simulink library "accelerometers"  (R2023b)
settings: Solver=VariableStepAuto  StartTime=0.0  StopTime=10.0  RelTol=1e-3
values from neighbouring files (symbols this model uses):
  acc_dynamic = 2*9.81    (= 19.62)    [sim_cfg.m]
  acc_freq = 100    [sim_cfg.m]
  acc_noise = 0.008*9.81    (= 0.07848)    [sim_cfg.m]
  acc_non_orthogonality = acc_axis_alignement*acc_non_orthogonality    [sim_cfg.m]
  gravity = 9.81+rand()*0.005    [sim_cfg.m]
libraries: simulink x1
settings Model: Creator=robin  LastModifiedBy=robin

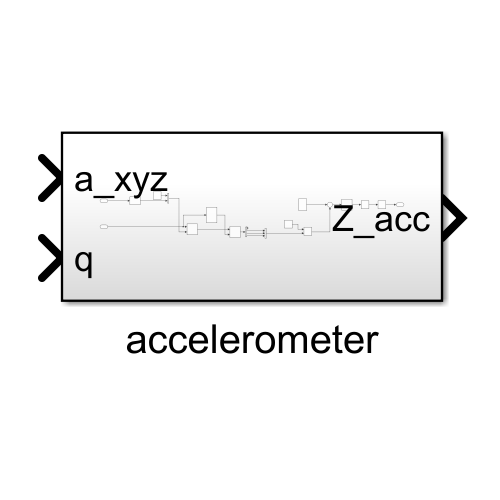
[thumbnail: Simulink's stored preview of the top-level diagram]
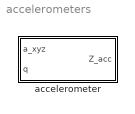
== system accelerometers ==
  accelerometer : Subsystem

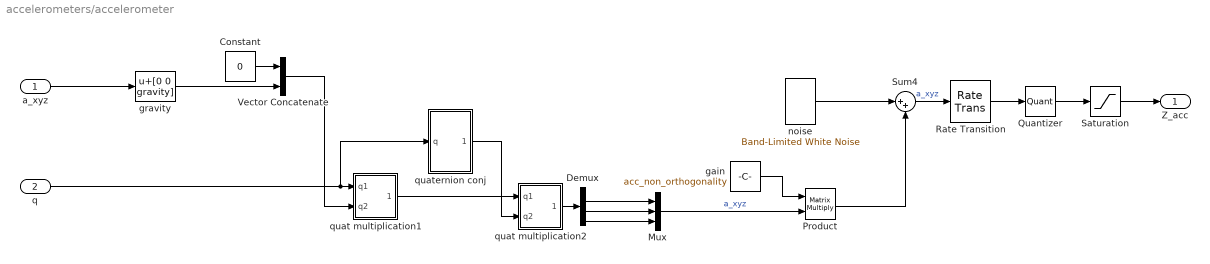
== system accelerometers/accelerometer ==
  a_xyz : Inport
  q : Inport  Port=2
  Constant : Constant  Value=0
  Demux : Demux
  Mux : Mux  Inputs=3
  Product : Product  Multiplication=Matrix(*)
  Quantizer : Quantizer  QuantizationInterval=acc_res
  Rate Transition : RateTransition  OutPortSampleTime=1/acc_freq
  Saturation : Saturate  UpperLimit=acc_dynamic  LowerLimit=-acc_dynamic
  Sum4 : Sum  Inputs=|++
  Vector Concatenate : Concatenate
  gain : Constant  Value=acc_non_orthogonality
  gravity : Bias  Bias=[0 0 gravity]  SaturateOnIntegerOverflow=off
  noise : simulink/Sources/Band-Limited White Noise  Cov=[2*(2*pi*acc_noise/acc_freq)^2 2*(2*pi*acc_noise/acc_freq)^2 2*(2*pi*acc_noise/acc_freq)^2]  Ts=1/acc_freq  seed=[randi(1000) randi(1000) randi(1000)]  VectorParams1D=off
  quat multiplication1 : Subsystem
  quat multiplication2 : Subsystem
  quaternion conj : Subsystem
  Z_acc : Outport
  wires:
  q/1 -> quat multiplication1/1(q1), quaternion conj/1(q)
  Sum4/1 -> Rate Transition/1  "a_xyz"
  Constant/1 -> Vector Concatenate/1
  Vector Concatenate/1 -> quat multiplication1/2(q2)
  gravity/1 -> Vector Concatenate/2
  quaternion conj/1(q conj) -> quat multiplication2/2(q2)
  quat multiplication1/1(q1*q2) -> quat multiplication2/1(q1)
  a_xyz/1 -> gravity/1
  quat multiplication2/1(q1*q2) -> Demux/1
  Demux/2 -> Mux/1
  Demux/3 -> Mux/2
  Demux/4 -> Mux/3
  gain/1 -> Product/1
  noise/1 -> Sum4/1
  Mux/1 -> Product/2  "a_xyz"
  Saturation/1 -> Z_acc/1
  Rate Transition/1 -> Quantizer/1
  Quantizer/1 -> Saturation/1
  Product/1 -> Sum4/2

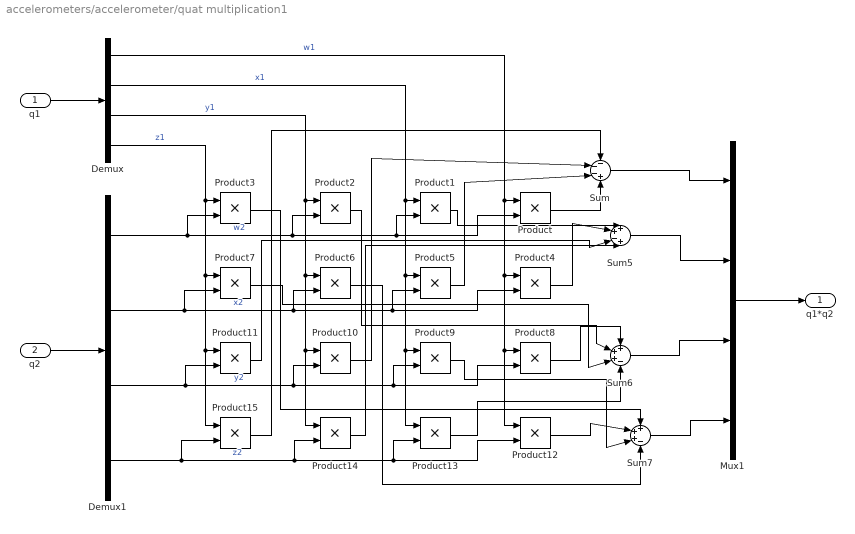
== system accelerometers/accelerometer/quat multiplication1 ==
  q1 : Inport
  q2 : Inport  Port=2
  Demux : Demux
  Demux1 : Demux
  Mux1 : Mux
  Product{,1..15} (16 alike) : Product
  Sum : Sum  Inputs=---+
  Sum5 : Sum  Inputs=++-+
  Sum6 : Sum  Inputs=+++-
  Sum7 : Sum  Inputs=+++-
  q1*q2 : Outport
  wires:
  Sum5/1 -> Mux1/2
  Product/1 -> Sum/4
  Product9/1 -> Sum7/3
  Demux/1 -> Product12/1, Product8/1, Product4/1, Product/1  "w1"
  Demux1/3 -> Product8/2, Product9/2, Product10/2, Product11/2  "y2"
  Demux/2 -> Product13/1, Product9/1, Product5/1, Product1/1  "x1"
  Product6/1 -> Sum7/4
  Product4/1 -> Sum5/2
  Demux1/1 -> Product/2, Product1/2, Product2/2, Product3/2  "w2"
  Sum/1 -> Mux1/1
  Product3/1 -> Sum7/1
  Product15/1 -> Sum/1
  Product1/1 -> Sum5/1
  Product2/1 -> Sum6/2
  Demux/4 -> Product15/1, Product11/1, Product7/1, Product3/1  "z1"
  Sum6/1 -> Mux1/3
  Demux1/2 -> Product4/2, Product5/2, Product6/2, Product7/2  "x2"
  Demux1/4 -> Product12/2, Product13/2, Product14/2, Product15/2  "z2"
  Product14/1 -> Sum5/4
  Mux1/1 -> q1*q2/1
  Sum7/1 -> Mux1/4
  Demux/3 -> Product14/1, Product10/1, Product6/1, Product2/1  "y1"
  Product13/1 -> Sum6/4
  Product8/1 -> Sum6/1
  q2/1 -> Demux1/1
  q1/1 -> Demux/1
  Product11/1 -> Sum5/3
  Product7/1 -> Sum6/3
  Product10/1 -> Sum/2
  Product5/1 -> Sum/3
  Product12/1 -> Sum7/2

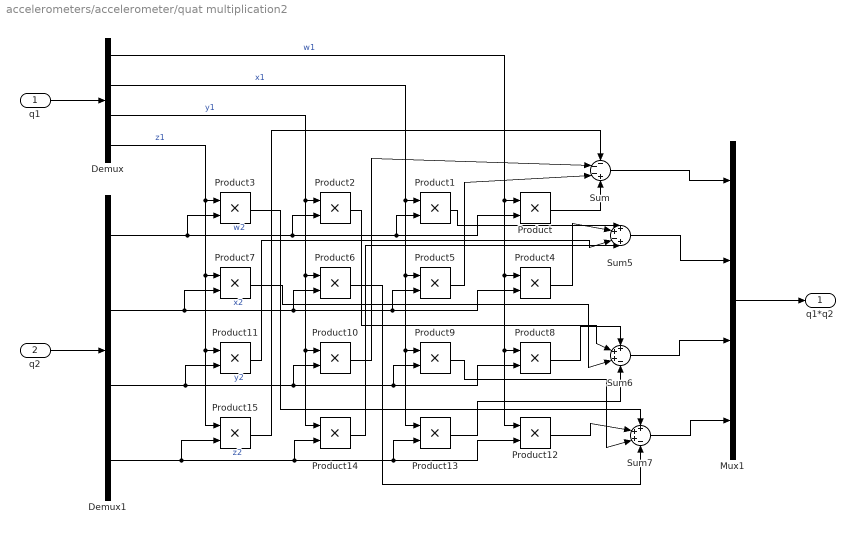
== system accelerometers/accelerometer/quat multiplication2 ==
  q1 : Inport
  q2 : Inport  Port=2
  Demux : Demux
  Demux1 : Demux
  Mux1 : Mux
  Product{,1..15} (16 alike) : Product
  Sum : Sum  Inputs=---+
  Sum5 : Sum  Inputs=++-+
  Sum6 : Sum  Inputs=+++-
  Sum7 : Sum  Inputs=+++-
  q1*q2 : Outport
  wires:
  Sum5/1 -> Mux1/2
  Product/1 -> Sum/4
  Product9/1 -> Sum7/3
  Demux/1 -> Product12/1, Product8/1, Product4/1, Product/1  "w1"
  Demux1/3 -> Product8/2, Product9/2, Product10/2, Product11/2  "y2"
  Demux/2 -> Product13/1, Product9/1, Product5/1, Product1/1  "x1"
  Product6/1 -> Sum7/4
  Product4/1 -> Sum5/2
  Demux1/1 -> Product/2, Product1/2, Product2/2, Product3/2  "w2"
  Sum/1 -> Mux1/1
  Product3/1 -> Sum7/1
  Product15/1 -> Sum/1
  Product1/1 -> Sum5/1
  Product2/1 -> Sum6/2
  Demux/4 -> Product15/1, Product11/1, Product7/1, Product3/1  "z1"
  Sum6/1 -> Mux1/3
  Demux1/2 -> Product4/2, Product5/2, Product6/2, Product7/2  "x2"
  Demux1/4 -> Product12/2, Product13/2, Product14/2, Product15/2  "z2"
  Product14/1 -> Sum5/4
  Mux1/1 -> q1*q2/1
  Sum7/1 -> Mux1/4
  Demux/3 -> Product14/1, Product10/1, Product6/1, Product2/1  "y1"
  Product13/1 -> Sum6/4
  Product8/1 -> Sum6/1
  q2/1 -> Demux1/1
  q1/1 -> Demux/1
  Product11/1 -> Sum5/3
  Product7/1 -> Sum6/3
  Product10/1 -> Sum/2
  Product5/1 -> Sum/3
  Product12/1 -> Sum7/2

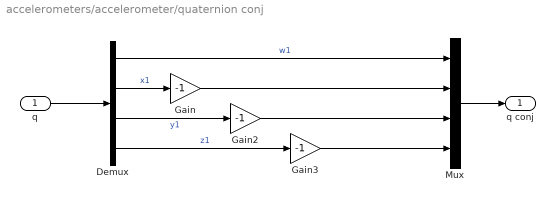
== system accelerometers/accelerometer/quaternion conj ==
  q : Inport
  Demux : Demux
  Gain : Gain  Gain=-1
  Gain2 : Gain  Gain=-1
  Gain3 : Gain  Gain=-1
  Mux : Mux
  q conj : Outport
  wires:
  Gain2/1 -> Mux/3
  Demux/3 -> Gain2/1  "y1"
  Demux/1 -> Mux/1  "w1"
  Gain3/1 -> Mux/4
  Demux/4 -> Gain3/1  "z1"
  q/1 -> Demux/1
  Mux/1 -> q conj/1
  Demux/2 -> Gain/1  "x1"
  Gain/1 -> Mux/2
